simulink library "pne_pne3d_generic_std"  (R2016a)
settings: Solver=VariableStepAuto  StartTime=0.0  StopTime=10.0  RelTol=1e-3
undefined symbols (not defined in the file): sMP
(part 4 of 7)

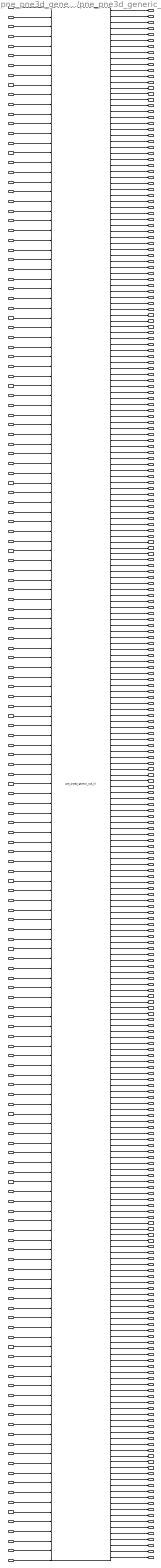
== system pne_pne3d_generic_std/pne_pne3d_generic_std ==
  ebs_AdditionalAxle_left_pDmd : Inport
  ebs_AdditionalAxle_left_setABS : Inport  Port=2
  ebs_AdditionalAxle_right_pDmd : Inport  Port=3
  ebs_AdditionalAxle_right_setABS : Inport  Port=4
  ebs_ESCsens_y_acceleration : Inport  Port=5
  ebs_FrontAxle_left_pDmd : Inport  Port=6
  ebs_FrontAxle_left_setABS : Inport  Port=7
  ebs_FrontAxle_right_pDmd : Inport  Port=8
  ebs_FrontAxle_right_setABS : Inport  Port=9
  ebs_RearAxle_left_pDmd : Inport  Port=10
  ebs_RearAxle_left_setABS : Inport  Port=11
  ebs_RearAxle_right_pDmd : Inport  Port=12
  ebs_RearAxle_right_setABS : Inport  Port=13
  ebs_sBSP_stABSInValve_Addl_Left : Inport  Port=14
  ebs_sBSP_stABSInValve_Addl_Right : Inport  Port=15
  ebs_sBSP_stABSInValve_Front_Left : Inport  Port=16
  ebs_sBSP_stABSInValve_Front_Right : Inport  Port=17
  ebs_sBSP_stABSInValve_RCMax_Front : Inport  Port=18
  ebs_sBSP_stABSInValve_RCMax_Rear : Inport  Port=19
  ebs_sBSP_stABSInValve_Rear_Left : Inport  Port=20
  ebs_sBSP_stABSInValve_Rear_Right : Inport  Port=21
  ebs_sBSP_stABSOutValve_Addl_Left : Inport  Port=22
  ebs_sBSP_stABSOutValve_Addl_Right : Inport  Port=23
  ebs_sBSP_stABSOutValve_Front_Left : Inport  Port=24
  ebs_sBSP_stABSOutValve_Front_Right : Inport  Port=25
  ebs_sBSP_stABSOutValve_RCMax_Front : Inport  Port=26
  ebs_sBSP_stABSOutValve_RCMax_Rear : Inport  Port=27
  ebs_sBSP_stABSOutValve_Rear_Left : Inport  Port=28
  ebs_sBSP_stABSOutValve_Rear_Right : Inport  Port=29
  ebs_sBSP_stAPCVBuValve : Inport  Port=30
  ebs_sBSP_stAPCVInValve : Inport  Port=31
  ebs_sBSP_stAPCVOutValve : Inport  Port=32
  ebs_sBSP_stAtcCutOffValve : Inport  Port=33
  ebs_sBSP_stAxmoBuValve : Inport  Port=34
  ebs_sBSP_stAxmoInValve_Rear_Left : Inport  Port=35
  ebs_sBSP_stAxmoInValve_Rear_Right : Inport  Port=36
  ebs_sBSP_stAxmoOutValve_Rear_Left : Inport  Port=37
  ebs_sBSP_stAxmoOutValve_Rear_Right : Inport  Port=38
  ebs_sBSP_stCMaxBuValve : Inport  Port=39
  ebs_sBSP_stCMaxInValve_Rear_Left : Inport  Port=40
  ebs_sBSP_stCMaxInValve_Rear_Right : Inport  Port=41
  ebs_sBSP_stCMaxOutValve_Rear_Left : Inport  Port=42
  ebs_sBSP_stCMaxOutValve_Rear_Right : Inport  Port=43
  ebs_sBSP_stRCMaxInValve_Front : Inport  Port=44
  ebs_sBSP_stRCMaxInValve_Rear : Inport  Port=45
  ebs_sBSP_stRCMaxOutValve_Front : Inport  Port=46
  ebs_sBSP_stRCMaxOutValve_Rear : Inport  Port=47
  ebs_sBSP_stTCVBuValve : Inport  Port=48
  ebs_sBSP_stTCVInValve : Inport  Port=49
  ebs_sBSP_stTCVOutValve : Inport  Port=50
  ebs_sil_AAle_force : Inport  Port=51
  ebs_sil_AAle_vel : Inport  Port=52
  ebs_sil_AAri_force : Inport  Port=53
  ebs_sil_AAri_vel : Inport  Port=54
  ebs_sil_FAle_force : Inport  Port=55
  ebs_sil_FAle_vel : Inport  Port=56
  ebs_sil_FAri_force : Inport  Port=57
  ebs_sil_FAri_vel : Inport  Port=58
  ebs_sil_RAle_force : Inport  Port=59
  ebs_sil_RAle_vel : Inport  Port=60
  ebs_sil_RAri_force : Inport  Port=61
  ebs_sil_RAri_vel : Inport  Port=62
  ebs_st3by2_First : Inport  Port=63
  ebs_st3by2_Second : Inport  Port=64
  ebs_TCV_pDmd : Inport  Port=65
  Failure_electric_circuit_AA : Inport  Port=66
  Failure_electric_circuit_FA : Inport  Port=67
  Failure_electric_circuit_RA : Inport  Port=68
  Failure_pneumatic_circuit_FA : Inport  Port=69
  Failure_pneumatic_circuit_RA : Inport  Port=70
  pneAux_A1_Le_Rq : Inport  Port=71
  pneAux_A1_LoLi_Rq : Inport  Port=72
  pneAux_A1_Ri_Rq : Inport  Port=73
  pneAux_A2_Le_Rq : Inport  Port=74
  pneAux_A2_LoLi_Rq : Inport  Port=75
  pneAux_A2_Ri_Rq : Inport  Port=76
  pneAux_A3_Le_Rq : Inport  Port=77
  pneAux_A3_LoLi_Rq : Inport  Port=78
  pneAux_A3_Ri_Rq : Inport  Port=79
  pneAux_Axle1_load : Inport  Port=80
  pneAux_Axle2_load : Inport  Port=81
  pneAux_Axle3_load : Inport  Port=82
  pneAux_Axle4_load : Inport  Port=83
  pneAux_Drs_Rq : Inport  Port=84
  pneAux_EAPU_overrun : Inport  Port=85
  pneAux_pSoll_TCV_p43 : Inport  Port=86
  pneAux_pSollPkBrk : Inport  Port=87
  pneAux_TCV_pDmd_Front_Left : Inport  Port=88
  pneAux_TCV_pDmd_Front_Right : Inport  Port=89
  pneAux_TCV_pDmd_Rear_Left : Inport  Port=90
  pneAux_TCV_pDmd_Rear_Right : Inport  Port=91
  pneAux_trailerAxle1_left_stABSInValve : Inport  Port=92
  pneAux_trailerAxle1_left_stABSOutValve : Inport  Port=93
  pneAux_trailerAxle1_load : Inport  Port=94
  pneAux_trailerAxle1_right_stABSInValve : Inport  Port=95
  pneAux_trailerAxle1_right_stABSOutValve : Inport  Port=96
  pneAux_trailerAxle2_left_stABSInValve : Inport  Port=97
  pneAux_trailerAxle2_left_stABSOutValve : Inport  Port=98
  pneAux_trailerAxle2_load : Inport  Port=99
  pneAux_trailerAxle2_right_stABSInValve : Inport  Port=100
  pneAux_trailerAxle2_right_stABSOutValve : Inport  Port=101
  pneAux_trailerAxle3_left_stABSInValve : Inport  Port=102
  pneAux_trailerAxle3_left_stABSOutValve : Inport  Port=103
  pneAux_trailerAxle3_load : Inport  Port=104
  pneAux_trailerAxle3_right_stABSInValve : Inport  Port=105
  pneAux_trailerAxle3_right_stABSOutValve : Inport  Port=106
  env_air_frontVel : Inport  Port=107
  env_pressure : Inport  Port=108
  env_Temperature : Inport  Port=109
  pne_brk_AirCompressor_angAcc : Inport  Port=110
  pne_brk_AirCompressor_angPos : Inport  Port=111
  pne_brk_AirCompressor_angVel : Inport  Port=112
  pne_brk_AirConsumpEng_mdot : Inport  Port=113
  pne_brk_AirConsumpRet_mdot : Inport  Port=114
  pne_brk_AirConsumpTx_mdot : Inport  Port=115
  pne_brk_Axle1_left_angAcc : Inport  Port=116
  pne_brk_Axle1_left_angPos : Inport  Port=117
  pne_brk_Axle1_left_angVel : Inport  Port=118
  pne_brk_Axle1_right_angAcc : Inport  Port=119
  pne_brk_Axle1_right_angPos : Inport  Port=120
  pne_brk_Axle1_right_angVel : Inport  Port=121
  pne_brk_Axle2_left_angAcc : Inport  Port=122
  pne_brk_Axle2_left_angPos : Inport  Port=123
  pne_brk_Axle2_left_angVel : Inport  Port=124
  pne_brk_Axle2_right_angAcc : Inport  Port=125
  pne_brk_Axle2_right_angPos : Inport  Port=126
  pne_brk_Axle2_right_angVel : Inport  Port=127
  pne_brk_Axle3_left_angAcc : Inport  Port=128
  pne_brk_Axle3_left_angPos : Inport  Port=129
  pne_brk_Axle3_left_angVel : Inport  Port=130
  pne_brk_Axle3_right_angAcc : Inport  Port=131
  pne_brk_Axle3_right_angPos : Inport  Port=132
  pne_brk_Axle3_right_angVel : Inport  Port=133
  pne_brk_Axle4_left_angAcc : Inport  Port=134
  pne_brk_Axle4_left_angPos : Inport  Port=135
  pne_brk_Axle4_left_angVel : Inport  Port=136
  pne_brk_Axle4_right_angAcc : Inport  Port=137
  pne_brk_Axle4_right_angPos : Inport  Port=138
  pne_brk_Axle4_right_angVel : Inport  Port=139
  pne_brk_CompressorInlet_massfracH2O : Inport  Port=140
  pne_brk_CompressorInlet_pressure : Inport  Port=141
  pne_brk_CompressorInlet_Temperature : Inport  Port=142
  pne_brk_PowerBoost_mdot : Inport  Port=143
  pne_brk_TrailerAxle1_left_angAcc : Inport  Port=144
  pne_brk_TrailerAxle1_left_angPos : Inport  Port=145
  pne_brk_TrailerAxle1_left_angVel : Inport  Port=146
  pne_brk_TrailerAxle1_right_angAcc : Inport  Port=147
  pne_brk_TrailerAxle1_right_angPos : Inport  Port=148
  pne_brk_TrailerAxle1_right_angVel : Inport  Port=149
  pne_brk_TrailerAxle2_left_angAcc : Inport  Port=150
  pne_brk_TrailerAxle2_left_angPos : Inport  Port=151
  pne_brk_TrailerAxle2_left_angVel : Inport  Port=152
  pne_brk_TrailerAxle2_right_angAcc : Inport  Port=153
  pne_brk_TrailerAxle2_right_angPos : Inport  Port=154
  pne_brk_TrailerAxle2_right_angVel : Inport  Port=155
  pne_brk_TrailerAxle3_left_angAcc : Inport  Port=156
  pne_brk_TrailerAxle3_left_angPos : Inport  Port=157
  pne_brk_TrailerAxle3_left_angVel : Inport  Port=158
  pne_brk_TrailerAxle3_right_angAcc : Inport  Port=159
  pne_brk_TrailerAxle3_right_angPos : Inport  Port=160
  pne_brk_TrailerAxle3_right_angVel : Inport  Port=161
  pne_pne3d_generic_std_sf : S-Function  FunctionName=pne_pne3d_generic_std_sf  Parameters=s1 s2 p1 p2 p3 p4 p5 p6 p7 p8 p9 p10 p11 p12 p13 p14 p15 p16 p17 p18 p19 p20 p21 p22 p23 p24 p25 p26 p27 p28 p29 p30 p31 p32 p33 p34 p35 p36 p37 p38 p39 p40 p41 p42 p43 p44 p45 p46 p47 p48 p49 p50 p51 p52 p53 p54 p55 p56 p57 p58 p59 p60 p61 p62 p63 p64 p65 p66 p67 p68 p69 p70 p71 p72 p73 p74 p75 p76 p77 p78 p79 p80 p81 p82 p83 p84 p85 p86 p87 p88 p89 p90 p91 p92 p93 p94 p95 p96 p97 p98 p99 p100 p101 p102 p103 p104 p105 p106 p107 p108 p109 p110 p111 p112 p113 p114 p115 p116 p117 p118 p119 p120 p121 p122 p123 p124 p125 p126 p127 p128 p129 p130 p131 p132 p133 p134 p135 p136 p137 p138 p139 p140 p141 p142 p143 p144 p145 p146 p147 p148 p149 p150 p151 p152 p153 p154 p155 p156 p157 p158 p159 p160 p161 p162 p163 p164 p165 p166 p167 p168 p169 p170 p171 p172 p173 p174 p175 p176 p177 p178 p179 p180 p181 p182 p183 p184 p185 p186 p187 p188 p189 p190 p191 p192 p193 p194 p195 p196 p197 p198 p199 p200 p201 p202 p203 p204 p205 p206 p207 p208 p209 p210 p211 p212 p213 p214 p215 p216 p217 p218 p219 p220 p221 p222 p223 p224 p225 p226 p227 p228 p229 p230 p231 p232 p233 p234 p235 p236 p237 p238 p239 p240 p241 p242 p243 p244 p245 p246 p247 p248 p249 p250 p251 p252 p253 p254 p255 p256 p257 p258 p259 p260 p261 p262 p263 p264 p265 p266 p267 p268 p269 p270 p271 p272 p273 p274 p275 p276 p277 p278 p279 p280 p281 p282 p283 p284 p285 p286 p287 p288 p289 p290 p291 p292 p293 p294 p295 p296 p297 p298 p299 p300 p301 p302 p303 p304 p305 p306 p307 p308 p309 p310 p311 p312 p313 p314 p315 p316 p317 p318 p319 p320 p321 p322 p323 p324 p325 p326 p327 p328 p329 p330 p331 p332 p333 p334 p335 p336 p337 p338 p339 p340 p341 p342 p343 p344 p345 p346 p347 p348 p349 p350 p351 p352 p353 p354 p355 p356 p357 p358 p359 p360 p361 p362 p363 p364 p365 p366 p367 p368 p369 p370 p371 p372 p373 p374 p375 p376 p377 p378 p379 p380 p381 p382 p383 p384 p385 p386 p387 p388 p389 p390 p391 p392 p393 p394 p395 p396 p397 p398 p399 p400 p401 p402 p403 p404 p405 p406 p407 p408 p409 p410 p411 p412 p413 p414 p415 p416 p417 p418 p419 p420 p421 p422 p423 p424 p425 p426 p427 p428 p429 p430 p431 p432 p433 p434 p435 p436 p437 p438 p439 p440 p441 p442 p443 p444 p445 p446 p447 p448 p449 p450 p451 p452 p453 p454 p455 p456 p457 p458 p459 p460 p461 p462 p463 p464 p465 p466 p467 p468 p469 p470 p471 p472 p473 p474 p475 p476 p477 p478 p479 p480 p481 p482 p483 p484 p485 p486 p487 p488 p489 p490 p491 p492 p493 p494 p495 p496 p497 p498 p499 p500 p501 p502 p503 p504 p505 p506 p507 p508 p509 p510 p511 p512 p513 p514 p515 p516 p517 p518 p519 p520 p521 p522 p523 p524 p525 p526 p527 p528 p529 p530 p531 p532 p533 p534 p535 p536 p537 p538 p539 p540 p541 p542 p543 p544 p545 p546 p547 p548 p549 p550 p551 p552 p553 p554 p555 p556 p557 p558 p559 p560 p561 p562 p563 p564 p565 p566 p567 p568 p569 p570 p571 p572 p573 p574 p575 p576 p577 p578 p579 p580 p581 p582 p583 p584 p585 p586 p587 p588 p589 p590 p591 p592 p593 p594 p595 p596 p597 p598 p599 p600 p601 p602 p603 p604 p605 p606 p607 p608 p609 p610 p611 p612 p613 p614 p615 p616 p617 p618 p619 p620 p621 p622 p623 p624 p625 p626 p627 p628 p629 p630 p631 p632 p633 p634 p635 p636 p637 p638 p639 p640 p641 p642 p643 p644 p645 p646 p647 p648 p649 p650 p651 p652 p653 p654 p655 p656 p657 p658 p659 p660 p661 p662 p663 p664 p665 p666 p667 p668 p669 p670 p671 p672 p673 p674 p675 p676 p677 p678 p679 p680 p681 p682 p683 p684 p685 p686 p687 p688 p689 p690 p691 p692 p693 p694 p695 p696 p697 p698 p699 p700 p701 p702 p703 p704 p705 p706 p707 p708 p709 p710 p711 p712 p713 p714 p715 p716 p717 p718 p719 p720 p721 p722 p723 p724 p725 p726 p727 p728 p729 p730 p731 p732 p733 p734 p735 p736 p737 p738 p739 p740 p741 p742 p743 p744 p745 p746 p747 p748 p749 p750 p751 p752 p753 p754 p755 p756 p757 p758 p759 p760 p761 p762 p763 p764 p765 p766 p767 p768 p769 p770 p771 p772 p773 p774 p775 p776 p777 p778 p779 p780 p781 p782 p783 p784 p785 p786 p787 p788 p789 p790 p791 p792 p793 p794 p795 p796 p797 p798 p799 p800 p801 p802 p803 p804 p805 p806 p807 p808 p809 p810 p811 p812 p813 p814 p815 p816 p817 p818 p819 p820 p821 p822 p823 p824 p825 p826 p827 p828 p829 p830 p831 p832 p833 p834 p835 p836 p837 p838 p839 p840 p841 p842 p843 p844 p845 p846 p847 p848 p849 p850 p851 p852 p853 p854 p855 p856 p857  SFunctionModules=pne_pne3d_generic_std_sf_decl pne_pne3d_generic_std_sf_functions pne_pne3d_generic_std_sf_init pne_pne3d_generic_std_sf_initjac pne_pne3d_generic_std_sf_jac ITI_ArrayFunctions ITI_big_uint ITI_FixStep_pne_pne3d_generic_std_sf ITI_Functions ITI_LinSolver ITI_Memory ITI_NonLinSolver_pne_pne3d_generic_std_sf ITI_SFuncFixStepSolver_pne_pne3d_generic_std_sf ITI_SFuncHelper ModelicaUtilities snprintf c_aes ModelicaIO ModelicaMatIO ModelicaStandardTables ModelicaStandardTablesUsertab zlib  SFunctionDeploymentMode=off  EnableBusSupport=off  mask{s1=s1, s2=s2, initCmd='Parameters_pne_pne3d_generic_std_sf', p1=p1, p2=p2, p3=p3, p4=p4, p5=p5, p6=p6, p7=p7, p8=p8, p9=p9, p10=p10, p11=p11, p12=p12, p13=p13, p14=p14, p15=p15, p16=p16, p17=p17, p18=p18, p19=p19, p20=p20, p21=p21, p22=p22, p23=p23, p24=p24, p25=p25, p26=p26, p27=p27, p28=p28, p29=p29, p30=p30, p31=p31, p32=p32, p33=p33, p34=p34, p35=p35, p36=p36, p37=p37, p38=p38, p39=p39, p40=p40, p41=p41, p42=p42, p43=p43, p44=p44, p45=p45, p46=p46, p47=p47, p48=p48, p49=p49, p50=p50, p51=p51, p52=p52, p53=p53, p54=p54, p55=p55, p56=p56, p57=p57, p58=p58, p59=p59, p60=p60, p61=p61, p62=p62, p63=p63, p64=p64, p65=p65, p66=p66, p67=p67, p68=p68, p69=p69, p70=p70, p71=p71, p72=p72, p73=p73, p74=p74, p75=p75, p76=p76, p77=p77, p78=p78, p79=p79, p80=p80, p81=p81, p82=p82, p83=p83, p84=p84, p85=p85, p86=p86, p87=p87, p88=p88, p89=p89, p90=p90, p91=p91, p92=p92, p93=p93, p94=p94, p95=p95, p96=p96, p97=p97, p98=p98, p99=p99, p100=p100, p101=p101, p102=p102, p103=p103, p104=p104, p105=p105, p106=p106, p107=p107, p108=p108, p109=p109, p110=p110, p111=p111, p112=p112, p113=p113, p114=p114, p115=p115, p116=p116, p117=p117, p118=p118, p119=p119, p120=p120, p121=p121, p122=p122, p123=p123, p124=p124, p125=p125, p126=p126, p127=p127, p128=p128, p129=p129, p130=p130, p131=p131, p132=p132, p133=p133, p134=p134, p135=p135, p136=p136, p137=p137, p138=p138, p139=p139, p140=p140, p141=p141, p142=p142, p143=p143, p144=p144, p145=p145, p146=p146, p147=p147, p148=p148, p149=p149, p150=p150, p151=p151, p152=p152, p153=p153, p154=p154, p155=p155, p156=p156, p157=p157, p158=p158, p159=p159, p160=p160, p161=p161, p162=p162, p163=p163, p164=p164, p165=p165, p166=p166, p167=p167, p168=p168, p169=p169, p170=p170, p171=p171, p172=p172, p173=p173, p174=p174, p175=p175, p176=p176, p177=p177, p178=p178, p179=p179, p180=p180, p181=p181, p182=p182, p183=p183, p184=p184, p185=p185, p186=p186, p187=p187, p188=p188, p189=p189, p190=p190, p191=p191, p192=p192, p193=p193, p194=p194, p195=p195, p196=p196, p197=p197, p198=p198, p199=p199, p200=p200, p201=p201, p202=p202, p203=p203, p204=p204, p205=p205, p206=p206, p207=p207, p208=p208, p209=p209, p210=p210, p211=p211, p212=p212, p213=p213, p214=p214, p215=p215, p216=p216, p217=p217, p218=p218, p219=p219, p220=p220, p221=p221, p222=p222, p223=p223, p224=p224, p225=p225, p226=p226, p227=p227, p228=p228, p229=p229, p230=p230, p231=p231, p232=p232, p233=p233, p234=p234, p235=p235, p236=p236, p237=p237, p238=p238, p239=p239, p240=p240, p241=p241, p242=p242, p243=p243, p244=p244, p245=p245, p246=p246, p247=p247, p248=p248, p249=p249, p250=p250, p251=p251, p252=p252, p253=p253, p254=p254, p255=p255, p256=p256, p257=p257, p258=p258, p259=p259, p260=p260, p261=p261, p262=p262, p263=p263, p264=p264, p265=p265, p266=p266, p267=p267, p268=p268, p269=p269, p270=p270, p271=p271, p272=p272, p273=p273, p274=p274, p275=p275, p276=p276, p277=p277, p278=p278, p279=p279, p280=p280, p281=p281, p282=p282, p283=p283, p284=p284, p285=p285, p286=p286, p287=p287, p288=p288, p289=p289, p290=p290, p291=p291, p292=p292, p293=p293, p294=p294, p295=p295, p296=p296, p297=p297, p298=p298, p299=p299, p300=p300, p301=p301, p302=p302, p303=p303, p304=p304, p305=p305, p306=p306, p307=p307, p308=p308, p309=p309, p310=p310, p311=p311, p312=p312, p313=p313, p314=p314, p315=p315, p316=p316, p317=p317, p318=p318, p319=p319, p320=p320, p321=p321, p322=p322, p323=p323, p324=p324, p325=p325, p326=p326, p327=p327, p328=p328, p329=p329, p330=p330, p331=p331, p332=p332, p333=p333, p334=p334, p335=p335, p336=p336, p337=p337, p338=p338, p339=p339, p340=p340, p341=p341, p342=p342, p343=p343, p344=p344, p345=p345, p346=p346, p347=p347, p348=p348, p349=p349, p350=p350, p351=p351, p352=p352, p353=p353, p354=p354, p355=p355, p356=p356, p357=p357, p358=p358, p359=p359, p360=p360, p361=p361, p362=p362, p363=p363, p364=p364, p365=p365, p366=p366, p367=p367, p368=p368, p369=p369, p370=p370, p371=p371, p372=p372, p373=p373, p374=p374, p375=p375, p376=p376, p377=p377, p378=p378, p379=p379, p380=p380, p381=p381, p382=p382, p383=p383, p384=p384, p385=p385, p386=p386, p387=p387, p388=p388, p389=p389, p390=p390, p391=p391, p392=p392, p393=p393, p394=p394, p395=p395, p396=p396, p397=p397, p398=p398, p399=p399, p400=p400, p401=p401, p402=p402, p403=p403, p404=p404, p405=p405, p406=p406, p407=p407, p408=p408, p409=p409, p410=p410, p411=p411, p412=p412, p413=p413, p414=p414, p415=p415, p416=p416, p417=p417, p418=p418, p419=p419, p420=p420, p421=p421, p422=p422, p423=p423, p424=p424, p425=p425, p426=p426, p427=p427, p428=p428, p429=p429, p430=p430, p431=p431, p432=p432, p433=p433, p434=p434, p435=p435, p436=p436, p437=p437, p438=p438, p439=p439, p440=p440, p441=p441, p442=p442, p443=p443, p444=p444, p445=p445, p446=p446, p447=p447, p448=p448, p449=p449, p450=p450, p451=p451, p452=p452, p453=p453, p454=p454, p455=p455, p456=p456, p457=p457, p458=p458, p459=p459, p460=p460, p461=p461, p462=p462, p463=p463, p464=p464, p465=p465, p466=p466, p467=p467, p468=p468, p469=p469, p470=p470, p471=p471, p472=p472, p473=p473, p474=p474, p475=p475, p476=p476, p477=p477, p478=p478, p479=p479, p480=p480, p481=p481, p482=p482, p483=p483, p484=p484, p485=p485, p486=p486, p487=p487, p488=p488, p489=p489, p490=p490, p491=p491, p492=p492, p493=p493, p494=p494, p495=p495, p496=p496, p497=p497, p498=p498, p499=p499, p500=p500, p501=p501, p502=p502, p503=p503, p504=p504, p505=p505, p506=p506, p507=p507, p508=p508, p509=p509, p510=p510, p511=p511, p512=p512, p513=p513, p514=p514, p515=p515, p516=p516, p517=p517, p518=p518, p519=p519, p520=p520, p521=p521, p522=p522, p523=p523, p524=p524, p525=p525, p526=p526, p527=p527, p528=p528, p529=p529, p530=p530, p531=p531, p532=p532, p533=p533, p534=p534, p535=p535, p536=p536, p537=p537, p538=p538, p539=p539, p540=p540, p541=p541, p542=p542, p543=p543, p544=p544, p545=p545, p546=p546, p547=p547, p548=p548, p549=p549, p550=p550, p551=p551, p552=p552, p553=p553, p554=p554, p555=p555, p556=p556, p557=p557, p558=p558, p559=p559, p560=p560, p561=p561, p562=p562, p563=p563, p564=p564, p565=p565, p566=p566, p567=p567, p568=p568, p569=p569, p570=p570, p571=p571, p572=p572, p573=p573, p574=p574, p575=p575, p576=p576, p577=p577, p578=p578, p579=p579, p580=p580, p581=p581, p582=p582, p583=p583, p584=p584, p585=p585, p586=p586, p587=p587, p588=p588, p589=p589, p590=p590, p591=p591, p592=p592, p593=p593, p594=p594, p595=p595, p596=p596, p597=p597, p598=p598, p599=p599, p600=p600, p601=p601, p602=p602, p603=p603, p604=p604, p605=p605, p606=p606, p607=p607, p608=p608, p609=p609, p610=p610, p611=p611, p612=p612, p613=p613, p614=p614, p615=p615, p616=p616, p617=p617, p618=p618, p619=p619, p620=p620, p621=p621, p622=p622, p623=p623, p624=p624, p625=p625, p626=p626, p627=p627, p628=p628, p629=p629, p630=p630, p631=p631, p632=p632, p633=p633, p634=p634, p635=p635, p636=p636, p637=p637, p638=p638, p639=p639, p640=p640, p641=p641, p642=p642, p643=p643, p644=p644, p645=p645, p646=p646, p647=p647, p648=p648, p649=p649, p650=p650, p651=p651, p652=p652, p653=p653, p654=p654, p655=p655, p656=p656, p657=p657, p658=p658, p659=p659, p660=p660, p661=p661, p662=p662, p663=p663, p664=p664, p665=p665, p666=p666, p667=p667, p668=p668, p669=p669, p670=p670, p671=p671, p672=p672, p673=p673, p674=p674, p675=p675, p676=p676, p677=p677, p678=p678, p679=p679, p680=p680, p681=p681, p682=p682, p683=p683, p684=p684, p685=p685, p686=p686, p687=p687, p688=p688, p689=p689, p690=p690, p691=p691, p692=p692, p693=p693, p694=p694, p695=p695, p696=p696, p697=p697, p698=p698, p699=p699, p700=p700, p701=p701, p702=p702, p703=p703, p704=p704, p705=p705, p706=p706, p707=p707, p708=p708, p709=p709, p710=p710, p711=p711, p712=p712, p713=p713, p714=p714, p715=p715, p716=p716, p717=p717, p718=p718, p719=p719, p720=p720, p721=p721, p722=p722, p723=p723, p724=p724, p725=p725, p726=p726, p727=p727, p728=p728, p729=p729, p730=p730, p731=p731, p732=p732, p733=p733, p734=p734, p735=p735, p736=p736, p737=p737, p738=p738, p739=p739, p740=p740, p741=p741, p742=p742, p743=p743, p744=p744, p745=p745, p746=p746, p747=p747, p748=p748, p749=p749, p750=p750, p751=p751, p752=p752, p753=p753, p754=p754, p755=p755, p756=p756, p757=p757, p758=p758, p759=p759, p760=p760, p761=p761, p762=p762, p763=p763, p764=p764, p765=p765, p766=p766, p767=p767, p768=p768, p769=p769, p770=p770, p771=p771, p772=p772, p773=p773, p774=p774, p775=p775, p776=p776, p777=p777, p778=p778, p779=p779, p780=p780, p781=p781, p782=p782, p783=p783, p784=p784, p785=p785, p786=p786, p787=p787, p788=p788, p789=p789, p790=p790, p791=p791, p792=p792, p793=p793, p794=p794, p795=p795, p796=p796, p797=p797, p798=p798, p799=p799, p800=p800, p801=p801, p802=p802, p803=p803, p804=p804, p805=p805, p806=p806, p807=p807, p808=p808, p809=p809, p810=p810, p811=p811, p812=p812, p813=p813, p814=p814, p815=p815, p816=p816, p817=p817, p818=p818, p819=p819, p820=p820, p821=p821, p822=p822, p823=p823, p824=p824, p825=p825, p826=p826, p827=p827, p828=p828, p829=p829, p830=p830, p831=p831, p832=p832, p833=p833, p834=p834, p835=p835, p836=p836, p837=p837, p838=p838, p839=p839, p840=p840, p841=p841, p842=p842, p843=p843, p844=p844, p845=p845, p846=p846, p847=p847, p848=p848, p849=p849, p850=p850, p851=p851, p852=p852, p853=p853, p854=p854, p855=p855, p856=p856, p857=p857}
